simulink model "extract_features"  (R2015b)
settings: Solver=VariableStepAuto  StartTime=0.0  StopTime=1406  RelTol=1e-3
undefined symbols (not defined in the file or in its folder): Rec, SDTV
libraries: visionconversions x2, visionstatistics x1
settings Model: Creator=User  LastModifiedBy=FLM

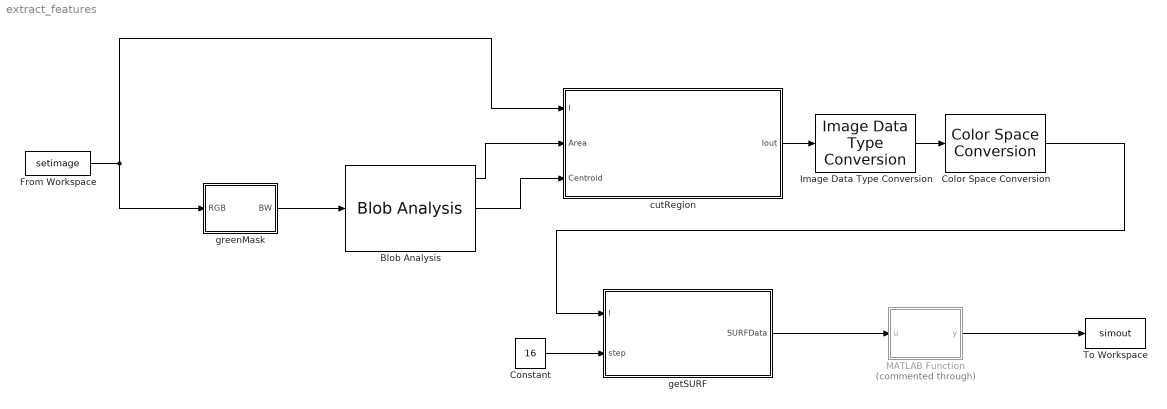
== system extract_features ==
  Blob Analysis : visionstatistics/Blob Analysis  Tag=vipblks_row_conv  area=on  centroid=on  bBox=on  majorAxis=off  minorAxis=off  angle=off  eccentricity=off  equivDiameterSq=off  extent=off  perimeter=off  maxBlobs=10  warnIfNumBlobsExceeded=on  isCount=off  useMinArea=off  minArea=0  useMaxArea=off  maxArea=intmax('uint32')  excludeBorderBlob=off  outDT=double  isOutVarDim=off  isFill=on  fillValues=-1  conn=8  isLabel=off  outputMode=Binary point scaling  outputWordLength=32  outputFracLength=16  firstCoeffMode=Binary point scaling  firstCoeffWordLength=16  firstCoeffFracLength=14  secondCoeffMode=Binary point scaling  secondCoeffWordLength=32  secondCoeffFracLength=16  accumMode=Binary point scaling  accumWordLength=32  accumFracLength=0  prodOutputMode=Binary point scaling  prodOutputWordLength=32  prodOutputFracLength=16  roundingMode=Floor  overflowMode=off
  Color Space Conversion : visionconversions/Color Space  Conversion  conversion=Obsolete  conversionActive=R'G'B' to HSV  wp_str=D65  rec=Rec. 601 (SDTV)  sys=1125/60/2:1  imagePorts=One multidimensional signal
  Constant : Constant  Value=16
  From Workspace : FromWorkspace  VariableName=setimage  SampleTime=1  OutputAfterFinalValue=Setting to zero
  Image Data Type Conversion : visionconversions/Image Data Type Conversion  outDT=double  isSigned=on  wordLen=16  numFracBits=0
  MATLAB Function : MATLAB Function  Commented=through  TreatAsAtomicUnit=on
  To Workspace : ToWorkspace  VariableName=simout  SampleTime=-1
  cutRegion : MATLAB Function  TreatAsAtomicUnit=on
  getSURF : MATLAB Function  TreatAsAtomicUnit=on
  greenMask : MATLAB Function  TreatAsAtomicUnit=on
  wires:
  greenMask/1(BW) -> Blob Analysis/1
  Blob Analysis/2 -> cutRegion/3(Centroid)
  Blob Analysis/1 -> cutRegion/2(Area)
  Constant/1 -> getSURF/2(step)
  From Workspace/1 -> cutRegion/1(I), greenMask/1(RGB)
  getSURF/1(SURFData) -> MATLAB Function/1(u)
  cutRegion/1(Iout) -> Image Data Type Conversion/1
  Image Data Type Conversion/1 -> Color Space Conversion/1
  Color Space Conversion/1 -> getSURF/1(I)
  MATLAB Function/1(y) -> To Workspace/1

== matlab function extract_features/cutRegion ==
  data: I input size=[240,320,3]; Area input; Centroid input; Iout output size=[160,160,3]
function Iout   = cutRegion(I,Area,Centroid)
%#codegen
Iout=uint8(zeros(160,160,3));
[Asort,index] = sort(Area,'descend');
cutSize = 160;
translation = [0,-20]; %move up 20 pixel
if Asort(1)<1000
    x = size(I,2)/2;
    y = size(I,1)/2;
else
    index = index(1);
    
    x = Centroid(index,1);
    y = Centroid(index,2);
end
x=round(x); y=round(y);
left =x-cutSize/2 + translation(1)+1;
right = x+cutSize/2 + translation(1);
top = y-cutSize/2 + translation(2)+1;
bottom = y+cutSize/2 + translation(2);
if left<1
    left = 1; right = cutSize;
end
if right>size(I,2)
    right = size(I,2);
    left = right - cutSize + 1;
end
if top < 1
    top = 1; bottom = cutSize;
end
if bottom > size(I,1)
    bottom = size(I,1);
    top = bottom - cutSize+1;
end
Iout(:)=I(top:bottom,left:right,1:3);
end

== matlab function extract_features/greenMask ==
  data: RGB input; BW output
function BW = greenMask(RGB)
%#codegen

%function [BW,maskedRGBImage] = createMask5(RGB)
%createMask  Threshold RGB image using auto-generated code from colorThresholder app.
%  [BW,MASKEDRGBIMAGE] = createMask(RGB) thresholds image RGB using
%  auto-generated code from the colorThresholder App. The colorspace and
%  minimum/maximum values for each channel of the colorspace were set in the
%  App and result in a binary mask BW and a composite image maskedRGBImage,
%  which shows the original RGB image values under the mask BW.

% Auto-generated by colorThresholder app on 01-Mar-2016
%------------------------------------------------------


% Convert RGB image to chosen color space
I = rgb2hsv(RGB);

% Define thresholds for channel 1 based on histogram settings
channel1Min = 0.187;
channel1Max = 0.514;

% Define thresholds for channel 2 based on histogram settings
channel2Min = 0.196;
channel2Max = 1.000;

% Define thresholds for channel 3 based on histogram settings
channel3Min = 0.000;
channel3Max = 0.650;

% Create mask based on chosen histogram thresholds
BW = (I(:,:,1) >= channel1Min ) & (I(:,:,1) <= channel1Max) & ...
    (I(:,:,2) >= channel2Min ) & (I(:,:,2) <= channel2Max) & ...
    (I(:,:,3) >= channel3Min ) & (I(:,:,3) <= channel3Max);

% Initialize output masked image based on input image.
%maskedRGBImage = RGB;

% Set background pixels where BW is false to zero.
%maskedRGBImage(repmat(~BW,[1 1 3])) = 0;

== matlab function extract_features/getSURF ==
  data: I input; SURFData output size=[1,22500]; step input
function SURFData   = getSURF_surf( I,step )
%#codegen

SURFData=zeros(1,22500);
SURFData(:) = getSURF_surf(I,step);
end

== matlab function extract_features/MATLAB Function ==
  data: u input; y output
function y = pca_to_score(u)
%#codegen
coeff = load('coeff_save.mat');
coeff= coeff.coeff;
y = zeros(1,349);
a=u*coeff;
y = a - repmat(mean(a),[size(a,1),1]);
